simulink model "IKTrajectoryControlExample"  (R2019b)
settings: Solver=ode3  StartTime=0.0  StopTime=40  FixedStep=Ts  RelTol=1e-3
PostLoadFcn:
  | sawyer = importrobot('sawyer.urdf');
  | sawyer.DataFormat = 'column';
  | 
  | I = imread('coins.png');
  | imageOrigin = [0.4,0.2,0.08];
  | scale = .0015;
model workspace (MAT data in the model file):
  I = [49 47 48 48 48 48 48 51 50 51 50 47 ... (73800 elements, 246x300)]
  Ts = 0.01
  filterConst = 0.08
  force_range = [0.8 0.9]
  imageOrigin = [0.4 0.2 0.08]
  initTargetPose = [-1  0  1.22464679915e-16  0.4; 0  1  0  0.2; -1.22464679915e-16  0  -1  0.28; 0  0  0  1]
  q0 = [0.422405030154; 0; -1.22880122285; -0.410622115963; 2.12106389539; 0.205505693545; 0.715545053124; 1.62245603969]
  robot = robotics.RigidBodyTree
  robot.TreeInternal = robotics.manip.internal.RigidBodyTree
  robot.TreeInternal.NumBodies = 6
  robot.TreeInternal.Base = robotics.manip.internal.RigidBody
  robot.TreeInternal.Base.Index = 0
  robot.TreeInternal.Base.NameInternal = 'base'
  robot.TreeInternal.Base.JointInternal = robotics.Joint
  robot.TreeInternal.Base.JointInternal.Type = 'fixed'
  robot.TreeInternal.Base.JointInternal.VelocityNumber = 0
  robot.TreeInternal.Base.JointInternal.PositionNumber = 0
  robot.TreeInternal.Base.JointInternal.MotionSubspace = [0; 0; 0; 0; 0; 0]
  robot.TreeInternal.Base.JointInternal.NameInternal = 'base_jnt'
  robot.TreeInternal.Base.ParentIndex = -1
  robot.TreeInternal.Base.ChildrenIndices = 1
  robot.TreeInternal.Base.MassInternal = 1
  robot.TreeInternal.Base.CenterOfMassInternal = [0 0 0]
  robot.TreeInternal.Base.InertiaInternal = [1  0  0; 0  1  0; 0  0  1]
  robot.TreeInternal.Base.SpatialInertia = [1  0  0  0  0  0; 0  1  0  0  0  0; 0  0  1  0  0  0; 0  0  0  1  0  0; 0  0  0  0  1  0; 0  0  0  0  0  1]
  robot.TreeInternal.Gravity = [0 0 0]
  robot.TreeInternal.Bodies{1} = robotics.manip.internal.RigidBody
  robot.TreeInternal.Bodies{1}.Index = 1
  robot.TreeInternal.Bodies{1}.NameInternal = 'body1'
  robot.TreeInternal.Bodies{1}.JointInternal = robotics.Joint
  robot.TreeInternal.Bodies{1}.JointInternal.Type = 'fixed'
  robot.TreeInternal.Bodies{1}.JointInternal.VelocityNumber = 0
  robot.TreeInternal.Bodies{1}.JointInternal.PositionNumber = 0
  robot.TreeInternal.Bodies{1}.JointInternal.MotionSubspace = [0; 0; 0; 0; 0; 0]
  robot.TreeInternal.Bodies{1}.JointInternal.InTree = 1
  robot.TreeInternal.Bodies{1}.JointInternal.ChildToJointTransform = [1  0  0  0; 0  1  0  0; 0  0  1  58; 0  0  0  1]
  robot.TreeInternal.Bodies{1}.JointInternal.NameInternal = 'jnt1'
  robot.TreeInternal.Bodies{1}.ParentIndex = 0
  robot.TreeInternal.Bodies{1}.ChildrenIndices = [0 1]
  robot.TreeInternal.Bodies{1}.MassInternal = 1
  robot.TreeInternal.Bodies{1}.CenterOfMassInternal = [0 0 0]
  robot.TreeInternal.Bodies{1}.InertiaInternal = [1  0  0; 0  1  0; 0  0  1]
  robot.TreeInternal.Bodies{1}.SpatialInertia = [1  0  0  0  0  0; 0  1  0  0  0  0; 0  0  1  0  0  0; 0  0  0  1  0  0; 0  0  0  0  1  0; 0  0  0  0  0  1]
  robot.TreeInternal.Bodies{2} = robotics.manip.internal.RigidBody
  robot.TreeInternal.Bodies{2}.Index = 2
  robot.TreeInternal.Bodies{2}.NameInternal = 'body2'
  robot.TreeInternal.Bodies{2}.JointInternal = robotics.Joint
  robot.TreeInternal.Bodies{2}.JointInternal.Type = 'revolute'
  robot.TreeInternal.Bodies{2}.JointInternal.VelocityNumber = 1
  robot.TreeInternal.Bodies{2}.JointInternal.PositionNumber = 1
  robot.TreeInternal.Bodies{2}.JointInternal.MotionSubspace = [0; 0; 1; 0; 0; 0]
  robot.TreeInternal.Bodies{2}.JointInternal.InTree = 1
  robot.TreeInternal.Bodies{2}.JointInternal.ChildToJointTransform = [1  0  0  0; 0  0.707106781187  -0.707106781187  0; 0  0.707106781187  0.707106781187  80; 0  0  0  1]
  robot.TreeInternal.Bodies{2}.JointInternal.NameInternal = 'jnt2'
  robot.TreeInternal.Bodies{2}.JointInternal.PositionLimitsInternal = [-3.14159265359 3.14159265359]
  robot.TreeInternal.Bodies{2}.JointInternal.JointAxisInternal = [0 0 1]
  robot.TreeInternal.Bodies{2}.ParentIndex = 1
  robot.TreeInternal.Bodies{2}.ChildrenIndices = [0 0 1]
  robot.TreeInternal.Bodies{2}.MassInternal = 1
  robot.TreeInternal.Bodies{2}.CenterOfMassInternal = [0 0 0]
  robot.TreeInternal.Bodies{2}.InertiaInternal = [1  0  0; 0  1  0; 0  0  1]
  robot.TreeInternal.Bodies{2}.SpatialInertia = [1  0  0  0  0  0; 0  1  0  0  0  0; 0  0  1  0  0  0; 0  0  0  1  0  0; 0  0  0  0  1  0; 0  0  0  0  0  1]
  robot.TreeInternal.Bodies{3} = robotics.manip.internal.RigidBody
  robot.TreeInternal.Bodies{3}.Index = 3
  robot.TreeInternal.Bodies{3}.NameInternal = 'body3'
  robot.TreeInternal.Bodies{3}.JointInternal = robotics.Joint
  robot.TreeInternal.Bodies{3}.JointInternal.Type = 'revolute'
  robot.TreeInternal.Bodies{3}.JointInternal.VelocityNumber = 1
  robot.TreeInternal.Bodies{3}.JointInternal.PositionNumber = 1
  robot.TreeInternal.Bodies{3}.JointInternal.MotionSubspace = [0; 0; 1; 0; 0; 0]
  robot.TreeInternal.Bodies{3}.JointInternal.InTree = 1
  robot.TreeInternal.Bodies{3}.JointInternal.ChildToJointTransform = [1  0  0  0; 0  6.12323399574e-17  -1  0; 0  1  6.12323399574e-17  135; 0  0  0  1]
  robot.TreeInternal.Bodies{3}.JointInternal.NameInternal = 'jnt3'
  robot.TreeInternal.Bodies{3}.JointInternal.PositionLimitsInternal = [-3.14159265359 3.14159265359]
  robot.TreeInternal.Bodies{3}.JointInternal.JointAxisInternal = [0 0 1]
  robot.TreeInternal.Bodies{3}.ParentIndex = 2
  robot.TreeInternal.Bodies{3}.ChildrenIndices = [0 0 0 1]
  robot.TreeInternal.Bodies{3}.MassInternal = 1
  robot.TreeInternal.Bodies{3}.CenterOfMassInternal = [0 0 0]
  robot.TreeInternal.Bodies{3}.InertiaInternal = [1  0  0; 0  1  0; 0  0  1]
  robot.TreeInternal.Bodies{3}.SpatialInertia = [1  0  0  0  0  0; 0  1  0  0  0  0; 0  0  1  0  0  0; 0  0  0  1  0  0; 0  0  0  0  1  0; 0  0  0  0  0  1]
  robot.TreeInternal.Bodies{4} = robotics.manip.internal.RigidBody
  robot.TreeInternal.Bodies{4}.Index = 4
  robot.TreeInternal.Bodies{4}.NameInternal = 'body4'
  robot.TreeInternal.Bodies{4}.JointInternal = robotics.Joint
  robot.TreeInternal.Bodies{4}.JointInternal.Type = 'revolute'
  robot.TreeInternal.Bodies{4}.JointInternal.VelocityNumber = 1
  robot.TreeInternal.Bodies{4}.JointInternal.PositionNumber = 1
  robot.TreeInternal.Bodies{4}.JointInternal.MotionSubspace = [0; 0; 1; 0; 0; 0]
  robot.TreeInternal.Bodies{4}.JointInternal.InTree = 1
  robot.TreeInternal.Bodies{4}.JointInternal.ChildToJointTransform = [1  0  0  0; 0  0.707106781187  0.707106781187  0; 0  -0.707106781187  0.707106781187  147; 0  0  0  1]
  robot.TreeInternal.Bodies{4}.JointInternal.NameInternal = 'jnt4'
  robot.TreeInternal.Bodies{4}.JointInternal.PositionLimitsInternal = [-3.14159265359 3.14159265359]
  robot.TreeInternal.Bodies{4}.JointInternal.JointAxisInternal = [0 0 1]
  robot.TreeInternal.Bodies{4}.ParentIndex = 3
  robot.TreeInternal.Bodies{4}.ChildrenIndices = [0 0 0 0 1]
  robot.TreeInternal.Bodies{4}.MassInternal = 1
  robot.TreeInternal.Bodies{4}.CenterOfMassInternal = [0 0 0]
  robot.TreeInternal.Bodies{4}.InertiaInternal = [1  0  0; 0  1  0; 0  0  1]
  robot.TreeInternal.Bodies{4}.SpatialInertia = [1  0  0  0  0  0; 0  1  0  0  0  0; 0  0  1  0  0  0; 0  0  0  1  0  0; 0  0  0  0  1  0; 0  0  0  0  0  1]
  robot.TreeInternal.Bodies{5} = robotics.manip.internal.RigidBody
  robot.TreeInternal.Bodies{5}.Index = 5
  robot.TreeInternal.Bodies{5}.NameInternal = 'body5'
  robot.TreeInternal.Bodies{5}.JointInternal = robotics.Joint
  robot.TreeInternal.Bodies{5}.JointInternal.Type = 'fixed'
  robot.TreeInternal.Bodies{5}.JointInternal.VelocityNumber = 0
  robot.TreeInternal.Bodies{5}.JointInternal.PositionNumber = 0
  robot.TreeInternal.Bodies{5}.JointInternal.MotionSubspace = [0; 0; 0; 0; 0; 0]
  robot.TreeInternal.Bodies{5}.JointInternal.InTree = 1
  robot.TreeInternal.Bodies{5}.JointInternal.ChildToJointTransform = [1  0  0  0; 0  6.12323399574e-17  -1  0; 0  1  6.12323399574e-17  30; 0  0  0  1]
  robot.TreeInternal.Bodies{5}.JointInternal.NameInternal = 'jnt5'
  robot.TreeInternal.Bodies{5}.ParentIndex = 4
  robot.TreeInternal.Bodies{5}.ChildrenIndices = [0 0 0 0 0 1]
  robot.TreeInternal.Bodies{5}.MassInternal = 1
  robot.TreeInternal.Bodies{5}.CenterOfMassInternal = [0 0 0]
  robot.TreeInternal.Bodies{5}.InertiaInternal = [1  0  0; 0  1  0; 0  0  1]
  robot.TreeInternal.Bodies{5}.SpatialInertia = [1  0  0  0  0  0; 0  1  0  0  0  0; 0  0  1  0  0  0; 0  0  0  1  0  0; 0  0  0  0  1  0; 0  0  0  0  0  1]
  robot.TreeInternal.Bodies{6} = robotics.manip.internal.RigidBody
  robot.TreeInternal.Bodies{6}.Index = 6
  robot.TreeInternal.Bodies{6}.NameInternal = 'body6'
  robot.TreeInternal.Bodies{6}.JointInternal = robotics.Joint
  robot.TreeInternal.Bodies{6}.JointInternal.Type = 'fixed'
  robot.TreeInternal.Bodies{6}.JointInternal.VelocityNumber = 0
  robot.TreeInternal.Bodies{6}.JointInternal.PositionNumber = 0
  robot.TreeInternal.Bodies{6}.JointInternal.MotionSubspace = [0; 0; 0; 0; 0; 0]
  robot.TreeInternal.Bodies{6}.JointInternal.InTree = 1
  robot.TreeInternal.Bodies{6}.JointInternal.ChildToJointTransform = [1  0  0  0; 0  1  0  0; 0  0  1  40; 0  0  0  1]
  robot.TreeInternal.Bodies{6}.JointInternal.NameInternal = 'jnt6'
  robot.TreeInternal.Bodies{6}.ParentIndex = 5
  robot.TreeInternal.Bodies{6}.ChildrenIndices = [0 0 0 0 0]
  robot.TreeInternal.Bodies{6}.MassInternal = 1
  robot.TreeInternal.Bodies{6}.CenterOfMassInternal = [0 0 0]
  robot.TreeInternal.Bodies{6}.InertiaInternal = [1  0  0; 0  1  0; 0  0  1]
  robot.TreeInternal.Bodies{6}.SpatialInertia = [1  0  0  0  0  0; 0  1  0  0  0  0; 0  0  1  0  0  0; 0  0  0  1  0  0; 0  0  0  0  1  0; 0  0  0  0  0  1]
  robot.TreeInternal.NumNonFixedBodies = 3
  robot.TreeInternal.PositionNumber = 3
  robot.TreeInternal.VelocityNumber = 3
  robot.TreeInternal.PositionDoFMap = [0  -1; 1  1; 2  2; 3  3; 0  -1; 0  -1]
  robot.TreeInternal.VelocityDoFMap = [0  -1; 1  1; 2  2; 3  3; 0  -1; 0  -1]
  robot.TreeInternal.MaxNumBodies = 6
  robot.TreeInternal.MaxNameLength = 200
  robot.TreeInternal.MaxJointPositionNumber = 7
  robot.TreeInternal.VisualizationInfo = robotics.manip.internal.VisualizationInfo
  robot.TreeInternal.VisualizationInfo.ShowTag = 'DO_NOT_EDIT_FmaL9'
  robot.TreeInternal.VisualizationInfo.EstimatedMaxReach = 415
  robot.TreeInternal.VisualizationInfo.IsMaxReachUpToDate = 1
  robot.TreeInternal.DataFormatInternal = 'struct'
  sawyer : robotics.RigidBodyTree (value not decoded)
  scale = 0.0015
  wayPoints = [0.4 0.4 0.4 0.4 0.4 0.4 0.4 0.4 0.4 0.4 0.4 0.4 ... (9846 elements, 1641x6)]
  weights = [1 1 1 1 1 1]
  weights1 = [1 1 1 1 1 1]
undefined symbols (not defined in the file or in its folder): Levenberg, Marquardt
libraries: robotmaniplib x6, simulink x5, robotcorelib x1
(part 1 of 2)
settings Model: OrderedModelArguments=off  Creator=The MathWorks, Inc.  LastModifiedBy=DXQ
settings DataIOCC: SaveFormat=StructureWithTime  ReturnWorkspaceOutputs=off
settings OptimizationCC: BlockReduction=off  BufferReuse=off
settings DebuggingCC: AlgebraicLoopMsg=none  UnconnectedInputMsg=none  UnconnectedOutputMsg=none  UnconnectedLineMsg=none  PregeneratedLibrarySubsystemCodeDiagnostic=none  UnderSpecifiedDimensionMsg=warning  ArithmeticOperatorsInVariantConditions=warning
settings SFSimCC: SimUseLocalCustomCode=off  CustomCodeUndefinedFunction=UseInterfaceOnly
settings RTWCC: RTWUseLocalCustomCode=off

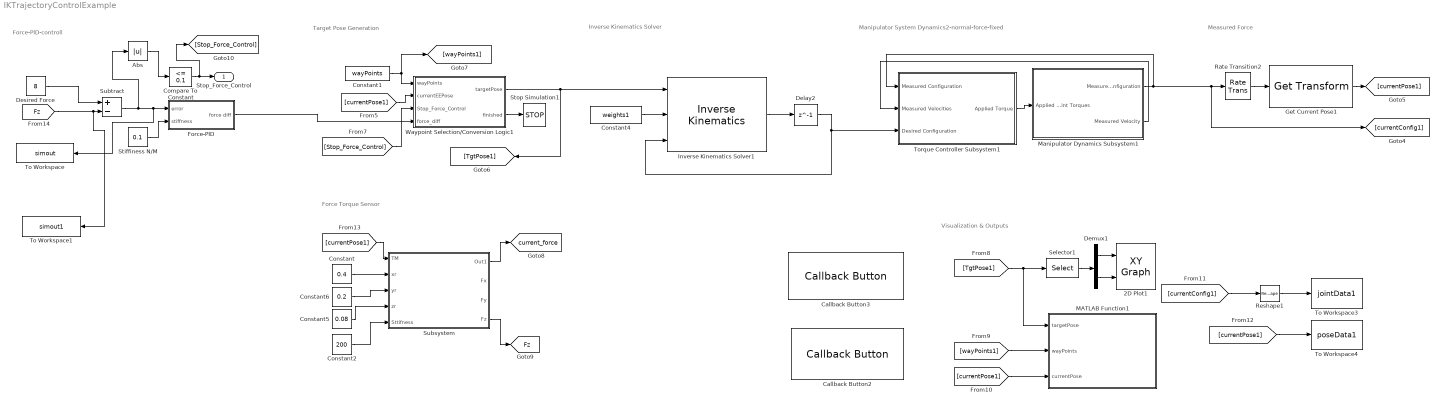
== system IKTrajectoryControlExample ==
  note: Force Torque Sensor
  note: Manipulator System Dynamics2-normal-force-fixed
  note: Measured Force
  note: Inverse Kinematics Solver
  note: Visualization & Outputs
  note: Target Pose Generation
  note: Force-PID-controll
  2D Plot1 : simulink/Sinks/XY Graph  xmin=.2  xmax=.9  ymin=0  ymax=.7  st=-1
  Abs : Abs
  Callback Button2 : CallbackButton  ButtonText=Show Image Processing Used for Waypoint Generation
      settings: ClickFcn=|
      | f1 = figure(1);
      | f1.Position = [158 253 953 335];
      | I1 = imread('coins.png');
      | I2 = imread('coinBoundaries.png');
      | 
      | subplot(1,2,1)
      | imshow(I1, 'Border', 'tight')
      | title('Original Image')
      | 
      | subplot(1,2,2)
      | imshow(I2, 'Border', 'tight')
      | title('Processed Image with Boundary Detection')
  Callback Button3 : CallbackButton  ButtonText=Visualize Model Output with Manipulator Mesh
      settings: ClickFcn=|
      | if exist('jointData', 'var')
      |     exampleHelperVisualizeIK(I, jointData, poseData, sawyer, imageOrigin, scale);
      | else
      |     sim(gcs)
      |     exampleHelperVisualizeIK(I, jointData, poseData, sawyer, imageOrigin, scale);
      | end
  Compare To Constant : simulink/Logic and Bit Operations/Compare To Constant  relop=<=  const=0.1  OutDataTypeStr=boolean
  Constant : Constant  Value=0.4
  Constant1 : Constant  Value=wayPoints
  Constant2 : Constant  Value=200
  Constant4 : Constant  Value=weights1
  Constant5 : Constant  Value=0.08
  Constant6 : Constant  Value=0.2
  Delay2 : Delay  DelayLength=1  InitialCondition=q0
  Demux1 : Demux  Outputs=2
  Desired Force : Constant  Value=8
  Force-PID : Subsystem  TreatAsAtomicUnit=on
  Get Current Pose1 : robotmaniplib/Get Transform  RigidBodyTree=sawyer  SourceBody=right_hand  TargetBody=base  SimulateUsing=Interpreted execution
      settings: SourceProductName=Robotics System Toolbox
  Inverse Kinematics Solver1 : robotmaniplib/Inverse Kinematics  RigidBodyTree=sawyer  EndEffector=right_hand  ShowInfo=off  SolverName=Levenberg-Marquardt  EnforceJointLimits=on  MaxIterations=1500  MaxTime=10  GradientTolerance=1e-7  SolutionTolerance=1e-5  StepTolerance=1e-14  ErrorChangeTolerance=1e-8  UseErrorDamping=on  DampingBias=0.0025  SimulateUsing=Interpreted execution
      settings: SourceProductName=Robotics System Toolbox
  MATLAB Function1 : MATLAB Function  TreatAsAtomicUnit=on  SystemSampleTime=.1
  Manipulator Dynamics Subsystem1 : Subsystem
  Rate Transition2 : RateTransition
  Reshape1 : Reshape
  Selector1 : Selector  NumberOfDimensions=2  IndexOptions=Index vector (dialog),Index vector (dialog)  Indices=[1 2],4  OutputSizes=1,1
  Stiffiness N/M : Constant  Value=0.1
  Stop Simulation1 : Stop
  Subsystem : Subsystem
  Subtract : Sum  Inputs=+-
  To Workspace : ToWorkspace  VariableName=simout  SaveFormat=Timeseries  SampleTime=-1
  To Workspace1 : ToWorkspace  VariableName=simout1  SaveFormat=Timeseries  SampleTime=-1
  To Workspace3 : ToWorkspace  VariableName=jointData1  SampleTime=-1
      settings: Save2DSignal=2-D array (concatenate along first dimension)
  To Workspace4 : ToWorkspace  VariableName=poseData1  SampleTime=-1
  Torque Controller Subsystem1 : Subsystem
  Waypoint Selection/Conversion Logic1 : Stateflow chart  TreatAsAtomicUnit=on
  "Stop_Force_Control " : Outport  VectorParamsAs1DForOutWhenUnconnected=off
  tag scope: Fz=global, current_force=global
  wires:
  Manipulator Dynamics Subsystem1/2(Measured Velocity) -> Torque Controller Subsystem1/2(Measured Velocities)
  Torque Controller Subsystem1/1(Applied Torque) -> Manipulator Dynamics Subsystem1/1(Applied Joint Torques)
  Rate Transition2/1 -> Get Current Pose1/1
  Manipulator Dynamics Subsystem1/1(Measured Configuration) -> Rate Transition2/1, [currentConfig1], Torque Controller Subsystem1/1(Measured Configuration)
  Get Current Pose1/1 -> [currentPose1]
  Inverse Kinematics Solver1/1 -> Delay2/1
  Delay2/1 -> Torque Controller Subsystem1/3(Desired Configuration), Inverse Kinematics Solver1/3
  [TgtPose1] -> Selector1/1, MATLAB Function1/1(targetPose)
  [currentConfig1] -> Reshape1/1
  [currentPose1] -> MATLAB Function1/3(currentPose)
  Demux1/2 -> 2D Plot1/2
  Selector1/1 -> Demux1/1
  Demux1/1 -> 2D Plot1/1
  Reshape1/1 -> To Workspace3/1
  [currentPose1] -> To Workspace4/1
  [wayPoints1] -> MATLAB Function1/2(wayPoints)
  Subsystem/1(Out1) -> [current_force]
  [currentPose1] -> Waypoint Selection/Conversion Logic1/2(currentEEPose)
  Waypoint Selection/Conversion Logic1/2(finished) -> Stop Simulation1/1
  Constant1/1 -> Waypoint Selection/Conversion Logic1/1(wayPoints), [wayPoints1]
  Waypoint Selection/Conversion Logic1/1(targetPose) -> [TgtPose1], Inverse Kinematics Solver1/1
  Constant4/1 -> Inverse Kinematics Solver1/2
  [Stop_Force_Control] -> Waypoint Selection/Conversion Logic1/3(Stop_Force_Control)
  Constant/1 -> Subsystem/2(xr)
  Constant6/1 -> Subsystem/3(yr)
  Constant5/1 -> Subsystem/4(zr)
  Constant2/1 -> Subsystem/5("Sttifness ")
  [currentPose1] -> Subsystem/1(TM)
  Compare To Constant/1 -> [Stop_Force_Control], "Stop_Force_Control "/1
  Desired Force/1 -> Subtract/1
  Stiffiness N/M/1 -> Force-PID/2(stiffness)
  Subtract/1 -> Abs/1, To Workspace/1, Force-PID/1(error)
  Force-PID/1(force diff) -> Waypoint Selection/Conversion Logic1/4(force_diff)
  [Fz] -> To Workspace1/1, Subtract/2
  Subsystem/4(Fz) -> [Fz]
  Abs/1 -> Compare To Constant/1
